simulink model "TorqueVectoringPathTrackingDriver"  (R2026b)
settings: Solver=FixedStepDiscrete  StopTime=1.0  FixedStep=TorqueVectoringControlSampleTime
undefined symbols (not defined in the file): TorqueVectoringEnableTV
settings Model: DataDictionary=VehicleData.sldd  Creator=Xu Dingyi  LastModifiedBy=29358
settings DebuggingCC: AlgebraicLoopMsg=error

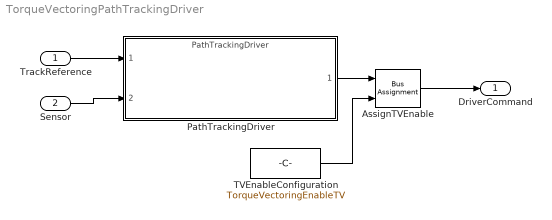
== system TorqueVectoringPathTrackingDriver ==
  TrackReference : Inport  OutDataTypeStr=Bus: TrackReferenceBus
  Sensor : Inport  Port=2  OutDataTypeStr=Bus: SensorBus
  AssignTVEnable : BusAssignment  AssignedSignals=EnableTV
  PathTrackingDriver : ModelReference  ModelNameDialog=PathTrackingDriver  ModelReferenceVersion=2.0
  TVEnableConfiguration : Constant  Value=TorqueVectoringEnableTV  OutDataTypeStr=boolean
  DriverCommand : Outport  OutDataTypeStr=Bus: DriverCommandBus
  wires:
  Sensor/1 -> PathTrackingDriver/2
  TrackReference/1 -> PathTrackingDriver/1
  AssignTVEnable/1 -> DriverCommand/1
  TVEnableConfiguration/1 -> AssignTVEnable/2
  PathTrackingDriver/1 -> AssignTVEnable/1
